simulink subsystem "darm_mechanics"  (R2021a)
settings: Solver=VariableStepAuto  StartTime=0.0  StopTime=10.0  RelTol=1e-3
undefined symbols (not defined in the file): darm, darm_knm, X, Y, Z
libraries: sm_lib x97, darm_library x77
(part 1 of 5)
settings Model: Creator=Daniel Adejumo  LastModifiedBy=Daniel Adejumo

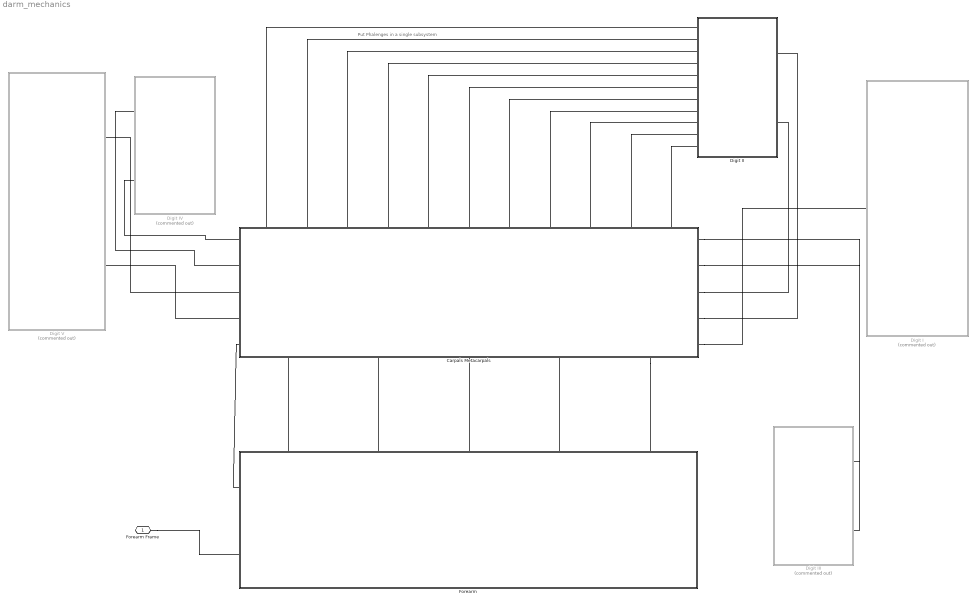
== system darm_mechanics ==
  note: Put Phalenges in a single subsystem
  Carpals Metacarpals : Subsystem
      settings: PortSchema="{\"entries\":[{\"content\":{\"sides\":[{\"content\":{\"connectorIds\":[\"LConn1\",\"LConn2\",\"LConn3\",\"LConn4\",\"LConn5\"]},\"type\":\"ConnectorPlacement.EquallySpacedRectSide\",\"uuid\":\"1bb88bb5-2f51-485d-a230-98e5c1753d25\"},{\"content\":{\"connectorIds\":[\"RConn1\",\"RConn2\",\"RConn3\",\"RConn4\",\"RConn5\"],\"side\":\"RIGHT\"},\"type\":\"ConnectorPlacement.EquallySpacedRectSide\",\"uuid\":\"55be408a-2070-4958-a81d-61010d6765a4\"},{\"content\":{\"connectorIds\":[\"LConn6\",\"LConn7\",\"LConn8\",\"LConn9\",\"LConn10\",\"LConn11\",\"LConn12\",\"LConn13\",\"LConn14\",\"LConn15\",\"LConn16\"],\"side\":\"TOP\"},\"type\":\"ConnectorPlacement.EquallySpacedRectSide\",\"uuid\":\"174f7df0-08cc-491e-9712-e123a58adeb3\"},{\"content\":{\"connectorIds\":[\"RConn6\",\"RConn7\",\"RConn8\",\"RConn9\",\"RConn10\"],\"side\":\"BOTTOM\"},\"type\":\"ConnectorPlacement.EquallySpacedRectSide\",\"uuid\":\"610f8ea9-4c2b-44d6-8efd-152cbdc7bfa9\"}]},\"type\":\"ConnectorPlacement.EquallySpacedConnector\",\"uuid\":\"f91d3c3d-350f-41e0-8fd3-766c28e2b75b\"}],\"packageUris\":[\"http://schema.mathworks.com/mf0/Connector/R2020b\"],\"version\":\"1.0\"}"
  Digit I : Subsystem  Commented=on
  Digit II : Subsystem
  Digit III : Subsystem  Commented=on
  Digit IV : Subsystem  Commented=on
  Digit V : Subsystem  Commented=on
  Forearm : Subsystem
      settings: PortSchema="{\"entries\":[{\"content\":{\"sides\":[{\"content\":{\"connectorIds\":[\"LConn1\",\"LConn2\"]},\"type\":\"ConnectorPlacement.EquallySpacedRectSide\",\"uuid\":\"5652e436-13d7-4977-ac7e-935b1a3f0729\"},{\"content\":{\"connectorIds\":[],\"side\":\"RIGHT\"},\"type\":\"ConnectorPlacement.EquallySpacedRectSide\",\"uuid\":\"721e98e9-19be-4402-ac40-382b694b4e6a\"},{\"content\":{\"connectorIds\":[\"LConn3\",\"LConn4\",\"LConn5\",\"LConn6\",\"LConn7\"],\"side\":\"TOP\"},\"type\":\"ConnectorPlacement.EquallySpacedRectSide\",\"uuid\":\"6b9e8076-ca0f-46eb-87d6-8c0e5d0c0dd4\"}]},\"type\":\"ConnectorPlacement.EquallySpacedConnector\",\"uuid\":\"9c8b8192-9cc9-4bae-a03f-e02120fb3373\"}],\"packageUris\":[\"http://schema.mathworks.com/mf0/Connector/R2020b\"],\"version\":\"1.0\"}"
  Forearm Frame : PMIOPort  Side=Left
  connections:
  Forearm Frame/RConn1 -- Forearm/LConn2
  Forearm/LConn1 -- Carpals Metacarpals/LConn5
  Carpals Metacarpals/RConn3 -- Digit II/RConn2
  Carpals Metacarpals/RConn4 -- Digit II/RConn1
  Carpals Metacarpals/RConn1 -- Digit III/RConn2
  Carpals Metacarpals/RConn2 -- Digit III/RConn1
  Carpals Metacarpals/LConn1 -- Digit IV/LConn2
  Carpals Metacarpals/LConn2 -- Digit IV/LConn1
  Carpals Metacarpals/LConn4 -- Digit V/RConn2
  Carpals Metacarpals/LConn3 -- Digit V/RConn1
  Carpals Metacarpals/RConn5 -- Digit I/RConn1
  Carpals Metacarpals/LConn6 -- Digit II/LConn1
  Carpals Metacarpals/LConn7 -- Digit II/LConn2
  Carpals Metacarpals/LConn8 -- Digit II/LConn3
  Carpals Metacarpals/LConn9 -- Digit II/LConn4
  Carpals Metacarpals/LConn10 -- Digit II/LConn5
  Carpals Metacarpals/LConn11 -- Digit II/LConn6
  Forearm/LConn3 -- Carpals Metacarpals/RConn6
  Forearm/LConn4 -- Carpals Metacarpals/RConn7
  Forearm/LConn5 -- Carpals Metacarpals/RConn8
  Carpals Metacarpals/LConn12 -- Digit II/LConn7
  Digit II/LConn8 -- Carpals Metacarpals/LConn13
  Carpals Metacarpals/LConn14 -- Digit II/LConn9
  Forearm/LConn6 -- Carpals Metacarpals/RConn9
  Carpals Metacarpals/LConn15 -- Digit II/LConn10
  Carpals Metacarpals/RConn10 -- Forearm/LConn7
  Carpals Metacarpals/LConn16 -- Digit II/LConn11

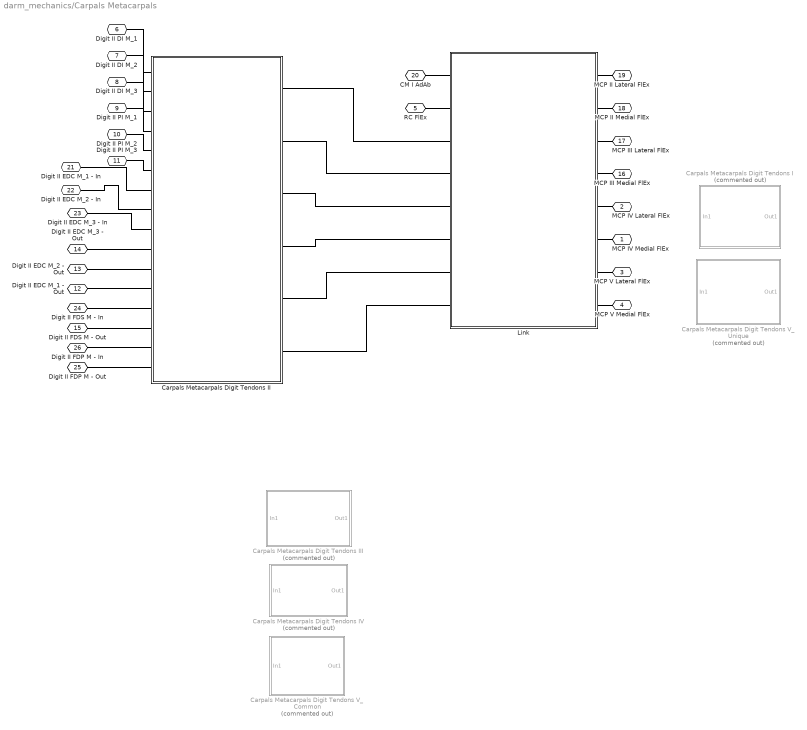
== system darm_mechanics/Carpals Metacarpals ==
  Carpals Metacarpals Digit Tendons I : Subsystem  Commented=on
  Carpals Metacarpals Digit Tendons II : Subsystem
  Carpals Metacarpals Digit Tendons III : Subsystem  Commented=on
  Carpals Metacarpals Digit Tendons IV : Subsystem  Commented=on
  Carpals Metacarpals Digit Tendons V_Common : Subsystem  Commented=on
  Carpals Metacarpals Digit Tendons V_Unique : Subsystem  Commented=on
  Link : Subsystem
  MCP IV Medial FlEx : PMIOPort  Side=Left
  MCP IV Lateral FlEx : PMIOPort  Port=2  Side=Left
  MCP V Lateral FlEx : PMIOPort  Port=3  Side=Left
  MCP V Medial FlEx : PMIOPort  Port=4  Side=Left
  RC FlEx : PMIOPort  Port=5  Side=Left
  Digit II DI M_1 : PMIOPort  Port=6  Side=Left
  Digit II DI M_2 : PMIOPort  Port=7  Side=Left
  Digit II DI M_3 : PMIOPort  Port=8  Side=Left
  Digit II PI M_1 : PMIOPort  Port=9  Side=Left
  Digit II PI M_2 : PMIOPort  Port=10  Side=Left
  Digit II PI M_3 : PMIOPort  Port=11  Side=Left
  Digit II EDC M_1 - Out : PMIOPort  Port=12  Side=Left
  Digit II EDC M_2 - Out : PMIOPort  Port=13  Side=Left
  Digit II EDC M_3 - Out : PMIOPort  Port=14  Side=Left
  Digit II FDS M - Out : PMIOPort  Port=15  Side=Left
  MCP III Medial FlEx : PMIOPort  Port=16  Side=Right
  MCP III Lateral FlEx : PMIOPort  Port=17  Side=Right
  MCP II Medial FlEx : PMIOPort  Port=18  Side=Right
  MCP II Lateral FlEx : PMIOPort  Port=19  Side=Right
  CM I AdAb : PMIOPort  Port=20  Side=Right
  Digit II EDC M_1 - In : PMIOPort  Port=21  Side=Right
  Digit II EDC M_2 - In : PMIOPort  Port=22  Side=Right
  Digit II EDC M_3 - In : PMIOPort  Port=23  Side=Right
  Digit II FDS M - In : PMIOPort  Port=24  Side=Right
  Digit II FDP M - Out : PMIOPort  Port=25  Side=Left
  Digit II FDP M - In : PMIOPort  Port=26  Side=Right
  connections:
  Digit II FDP M - In/RConn1 -- Carpals Metacarpals Digit Tendons II/LConn15
  Digit II FDP M - Out/RConn1 -- Carpals Metacarpals Digit Tendons II/LConn16
  Carpals Metacarpals Digit Tendons II/RConn6 -- Link/RConn8
  Carpals Metacarpals Digit Tendons II/RConn5 -- Link/RConn7
  Carpals Metacarpals Digit Tendons II/RConn4 -- Link/RConn6
  Digit II FDS M - Out/RConn1 -- Carpals Metacarpals Digit Tendons II/LConn14
  Digit II FDS M - In/RConn1 -- Carpals Metacarpals Digit Tendons II/LConn13
  Carpals Metacarpals Digit Tendons II/RConn3 -- Link/RConn5
  Digit II EDC M_1 - Out/RConn1 -- Carpals Metacarpals Digit Tendons II/LConn12
  Digit II EDC M_2 - Out/RConn1 -- Carpals Metacarpals Digit Tendons II/LConn11
  Digit II EDC M_3 - Out/RConn1 -- Carpals Metacarpals Digit Tendons II/LConn10
  Digit II EDC M_3 - In/RConn1 -- Carpals Metacarpals Digit Tendons II/LConn9
  Digit II EDC M_2 - In/RConn1 -- Carpals Metacarpals Digit Tendons II/LConn8
  Digit II EDC M_1 - In/RConn1 -- Carpals Metacarpals Digit Tendons II/LConn7
  Carpals Metacarpals Digit Tendons II/RConn2 -- Link/RConn4
  Digit II PI M_3/RConn1 -- Carpals Metacarpals Digit Tendons II/LConn6
  Digit II PI M_2/RConn1 -- Carpals Metacarpals Digit Tendons II/LConn5
  Digit II PI M_1/RConn1 -- Carpals Metacarpals Digit Tendons II/LConn4
  Digit II DI M_3/RConn1 -- Carpals Metacarpals Digit Tendons II/LConn3
  Digit II DI M_2/RConn1 -- Carpals Metacarpals Digit Tendons II/LConn2
  Digit II DI M_1/RConn1 -- Carpals Metacarpals Digit Tendons II/LConn1
  Carpals Metacarpals Digit Tendons II/RConn1 -- Link/RConn3
  CM I AdAb/RConn1 -- Link/RConn1
  Link/LConn8 -- MCP V Medial FlEx/RConn1
  Link/LConn7 -- MCP V Lateral FlEx/RConn1
  Link/LConn6 -- MCP IV Medial FlEx/RConn1
  Link/LConn5 -- MCP IV Lateral FlEx/RConn1
  Link/LConn4 -- MCP III Medial FlEx/RConn1
  Link/LConn3 -- MCP III Lateral FlEx/RConn1
  MCP II Medial FlEx/RConn1 -- Link/LConn2
  MCP II Lateral FlEx/RConn1 -- Link/LConn1
  RC FlEx/RConn1 -- Link/RConn2

== system darm_mechanics/Digit I ==
  Digit Links Assembly : Subsystem  AncestorBlock=darm_library/Digit Links Assembly  mask{digit=darm_knm.phalenges.digit_i}
      mask prompts: digit "Digit Struct"
      mask DialogControl DescGroupVar Prompt: Digit Links Assembly
      mask DialogControl DescTextVar Prompt: Assembles the phalanxes and joint shafts of a digit. Assembly spans from the proximal phalanx to the distal phalanx, excluding MCP Joint shafts.
  CM AdAb : PMIOPort  Side=Right
  connections:
  Digit Links Assembly/LConn4 -- CM AdAb/RConn1

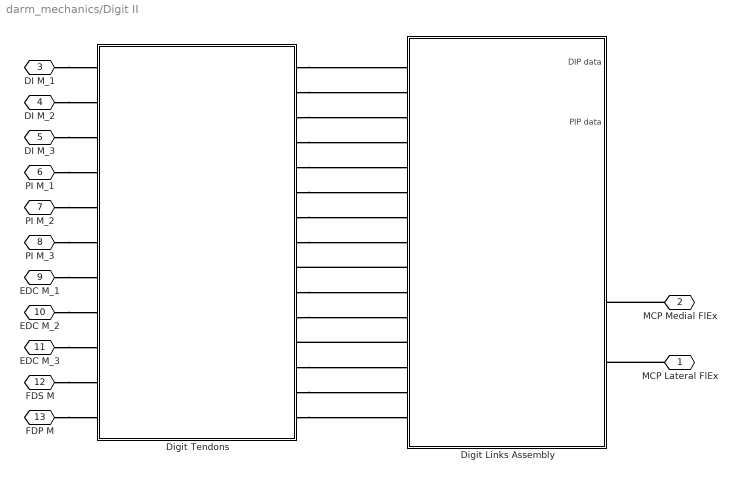
== system darm_mechanics/Digit II ==
  Digit Links Assembly : Subsystem  AncestorBlock=darm_library/Digit Links Assembly  mask{digit=darm.phalenges.digit_ii}
      mask prompts: digit "Digit Struct"
      mask DialogControl DescGroupVar Prompt: Digit Links Assembly
      mask DialogControl DescTextVar Prompt: Assembles the phalanxes and joint shafts of a digit. Assembly spans from the proximal phalanx to the distal phalanx, excluding MCP Joint shafts.
  Digit Tendons : Subsystem
  MCP Lateral FlEx : PMIOPort  Side=Right
  MCP Medial FlEx : PMIOPort  Port=2  Side=Right
  DI M_1 : PMIOPort  Port=3  Side=Left
  DI M_2 : PMIOPort  Port=4  Side=Left
  DI M_3 : PMIOPort  Port=5  Side=Left
  PI M_1 : PMIOPort  Port=6  Side=Left
  PI M_2 : PMIOPort  Port=7  Side=Left
  PI M_3 : PMIOPort  Port=8  Side=Left
  EDC M_1 : PMIOPort  Port=9  Side=Left
  EDC M_2 : PMIOPort  Port=10  Side=Left
  EDC M_3 : PMIOPort  Port=11  Side=Left
  FDS M : PMIOPort  Port=12  Side=Left
  FDP M : PMIOPort  Port=13  Side=Left
  connections:
  Digit Tendons/RConn15 -- Digit Links Assembly/LConn15
  Digit Tendons/RConn14 -- Digit Links Assembly/LConn14
  Digit Tendons/RConn1 -- Digit Links Assembly/LConn1
  FDP M/RConn1 -- Digit Tendons/LConn11
  Digit Tendons/RConn13 -- Digit Links Assembly/LConn13
  Digit Links Assembly/LConn12 -- Digit Tendons/RConn12
  FDS M/RConn1 -- Digit Tendons/LConn10
  Digit Tendons/RConn3 -- Digit Links Assembly/LConn3
  EDC M_3/RConn1 -- Digit Tendons/LConn9
  EDC M_2/RConn1 -- Digit Tendons/LConn8
  EDC M_1/RConn1 -- Digit Tendons/LConn7
  Digit Tendons/RConn8 -- Digit Links Assembly/LConn8
  Digit Tendons/RConn7 -- Digit Links Assembly/LConn7
  Digit Tendons/RConn11 -- Digit Links Assembly/LConn11
  PI M_3/RConn1 -- Digit Tendons/LConn6
  PI M_2/RConn1 -- Digit Tendons/LConn5
  PI M_1/RConn1 -- Digit Tendons/LConn4
  Digit Tendons/RConn10 -- Digit Links Assembly/LConn10
  Digit Links Assembly/LConn9 -- Digit Tendons/RConn9
  Digit Tendons/RConn5 -- Digit Links Assembly/LConn5
  DI M_3/RConn1 -- Digit Tendons/LConn3
  DI M_2/RConn1 -- Digit Tendons/LConn2
  Digit Tendons/RConn2 -- Digit Links Assembly/LConn2
  Digit Tendons/RConn4 -- Digit Links Assembly/LConn4
  DI M_1/RConn1 -- Digit Tendons/LConn1
  Digit Tendons/RConn6 -- Digit Links Assembly/LConn6
  MCP Lateral FlEx/RConn1 -- Digit Links Assembly/RConn4
  MCP Medial FlEx/RConn1 -- Digit Links Assembly/RConn3

== system darm_mechanics/Digit III ==
  Digit Links Assembly : Subsystem  AncestorBlock=darm_library/Digit Links Assembly  mask{digit=darm_knm.phalenges.digit_iii}
      mask prompts: digit "Digit Struct"
      mask DialogControl DescGroupVar Prompt: Digit Links Assembly
      mask DialogControl DescTextVar Prompt: Assembles the phalanxes and joint shafts of a digit. Assembly spans from the proximal phalanx to the distal phalanx, excluding MCP Joint shafts.
  MCP Lateral FlEx : PMIOPort  Side=Right
  MCP Medial FlEx : PMIOPort  Port=2  Side=Right
  connections:
  Digit Links Assembly/LConn4 -- MCP Lateral FlEx/RConn1
  Digit Links Assembly/LConn5 -- MCP Medial FlEx/RConn1

== system darm_mechanics/Digit IV ==
  Digit Links Assembly : Subsystem  AncestorBlock=darm_library/Digit Links Assembly  mask{digit=darm_knm.phalenges.digit_iv}
      mask prompts: digit "Digit Struct"
      mask DialogControl DescGroupVar Prompt: Digit Links Assembly
      mask DialogControl DescTextVar Prompt: Assembles the phalanxes and joint shafts of a digit. Assembly spans from the proximal phalanx to the distal phalanx, excluding MCP Joint shafts.
  MCP Lateral FlEx : PMIOPort  Side=Left
  MCP Medial FlEx : PMIOPort  Port=2  Side=Left
  connections:
  Digit Links Assembly/LConn4 -- MCP Lateral FlEx/RConn1
  Digit Links Assembly/LConn5 -- MCP Medial FlEx/RConn1

== system darm_mechanics/Digit V ==
  Digit Links Assembly : Subsystem  AncestorBlock=darm_library/Digit Links Assembly  mask{digit=darm_knm.phalenges.digit_v}
      mask prompts: digit "Digit Struct"
      mask DialogControl DescGroupVar Prompt: Digit Links Assembly
      mask DialogControl DescTextVar Prompt: Assembles the phalanxes and joint shafts of a digit. Assembly spans from the proximal phalanx to the distal phalanx, excluding MCP Joint shafts.
  MCP Lateral FlEx : PMIOPort  Side=Right
  MCP Medial FlEx : PMIOPort  Port=2  Side=Right
  connections:
  Digit Links Assembly/LConn5 -- MCP Medial FlEx/RConn1
  Digit Links Assembly/LConn4 -- MCP Lateral FlEx/RConn1

== system darm_mechanics/Forearm ==
  Forearm Digit Tendons II : Subsystem
  Link : Subsystem
  RC FlEx : PMIOPort  Side=Left
  Forearm Frame : PMIOPort  Port=2  Side=Left
  Digit II EDC M_1 : PMIOPort  Port=3  Side=Left
  Digit II EDC M_2 : PMIOPort  Port=4  Side=Left
  Digit II EDC M_3 : PMIOPort  Port=5  Side=Left
  Digit II FDS M : PMIOPort  Port=6  Side=Left
  Digit II FDP M : PMIOPort  Port=7  Side=Left
  connections:
  Digit II FDP M/RConn1 -- Forearm Digit Tendons II/LConn5
  Digit II FDS M/RConn1 -- Forearm Digit Tendons II/LConn4
  Digit II EDC M_1/RConn1 -- Forearm Digit Tendons II/LConn1
  Digit II EDC M_2/RConn1 -- Forearm Digit Tendons II/LConn2
  Digit II EDC M_3/RConn1 -- Forearm Digit Tendons II/LConn3
  Link/RConn1 -- Forearm Digit Tendons II/RConn1 -- RC FlEx/RConn1
  Forearm Digit Tendons II/RConn2 -- Forearm Frame/RConn1 -- Link/RConn2

== system darm_mechanics/Carpals Metacarpals/Carpals Metacarpals Digit Tendons I ==
  In1 : Inport
  Out1 : Outport
  wires:
  In1/1 -> Out1/1

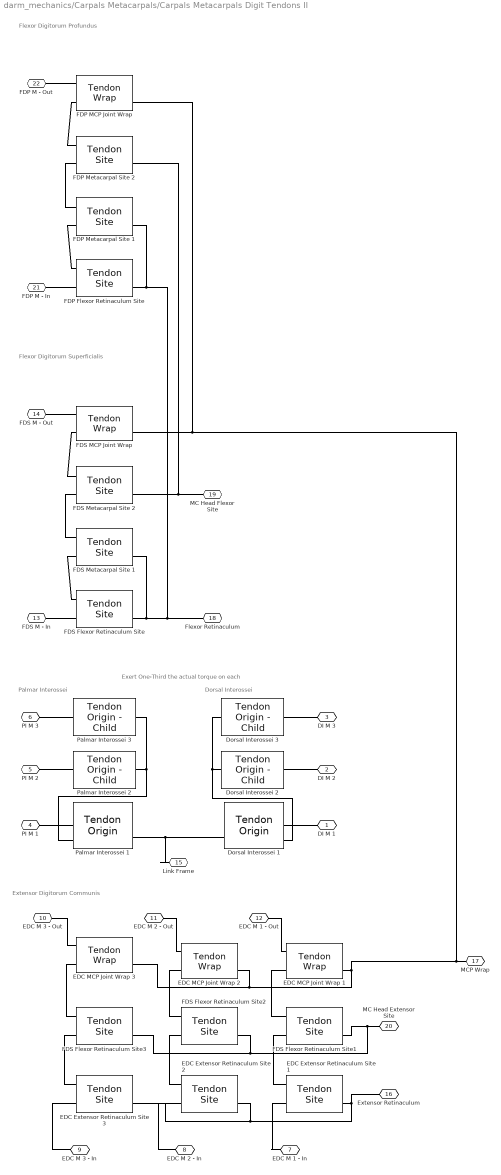
== system darm_mechanics/Carpals Metacarpals/Carpals Metacarpals Digit Tendons II ==
  note: Flexor Digitorum Profundus
  note: Palmar Interossei
  note: Exert One-Third the actual torque on each
  note: Dorsal Interossei
  note: Extensor Digitorum Communis
  note: Flexor Digitorum Superficialis
  Dorsal Interossei 1 : darm_library/Tendon Origin  muscle=darm.muscles.dorsal_interossei
  Dorsal Interossei 2 : darm_library/Tendon Origin - Child  muscle=darm.muscles.dorsal_interossei
  Dorsal Interossei 3 : darm_library/Tendon Origin - Child  muscle=darm.muscles.dorsal_interossei
  EDC Extensor Retinaculum Site 1 : darm_library/Tendon Site  muscle=darm.muscles.extensor_digitorum  site_index=1
  EDC Extensor Retinaculum Site 2 : darm_library/Tendon Site  muscle=darm.muscles.extensor_digitorum  site_index=1
  EDC Extensor Retinaculum Site 3 : darm_library/Tendon Site  muscle=darm.muscles.extensor_digitorum  site_index=1
  EDC MCP Joint Wrap 1 : darm_library/Tendon Wrap  muscle=darm.muscles.extensor_digitorum  wrap_index=2  flip=off
  EDC MCP Joint Wrap 2 : darm_library/Tendon Wrap  muscle=darm.muscles.extensor_digitorum  wrap_index=2  flip=off
  EDC MCP Joint Wrap 3 : darm_library/Tendon Wrap  muscle=darm.muscles.extensor_digitorum  wrap_index=2  flip=off
  FDP Flexor Retinaculum Site : darm_library/Tendon Site  muscle=darm.muscles.flexor_digitorum_profundus  site_index=1
  FDP MCP Joint Wrap : darm_library/Tendon Wrap  muscle=darm.muscles.flexor_digitorum_profundus  wrap_index=2  flip=on
  FDP Metacarpal Site 1 : darm_library/Tendon Site  muscle=darm.muscles.flexor_digitorum_profundus  site_index=3
  FDP Metacarpal Site 2 : darm_library/Tendon Site  muscle=darm.muscles.flexor_digitorum_profundus  site_index=5
  FDS Flexor Retinaculum Site : darm_library/Tendon Site  muscle=darm.muscles.flexor_digitorum_superficialis  site_index=1
  FDS Flexor Retinaculum Site1 : darm_library/Tendon Site  muscle=darm.muscles.extensor_digitorum  site_index=3
  FDS Flexor Retinaculum Site2 : darm_library/Tendon Site  muscle=darm.muscles.extensor_digitorum  site_index=3
  FDS Flexor Retinaculum Site3 : darm_library/Tendon Site  muscle=darm.muscles.extensor_digitorum  site_index=3
  FDS MCP Joint Wrap : darm_library/Tendon Wrap  muscle=darm.muscles.flexor_digitorum_superficialis  wrap_index=2  flip=on
  FDS Metacarpal Site 1 : darm_library/Tendon Site  muscle=darm.muscles.flexor_digitorum_superficialis  site_index=3
  FDS Metacarpal Site 2 : darm_library/Tendon Site  muscle=darm.muscles.flexor_digitorum_superficialis  site_index=5
  Palmar Interossei 1 : darm_library/Tendon Origin  muscle=darm.muscles.palmar_interossei
  Palmar Interossei 2 : darm_library/Tendon Origin - Child  muscle=darm.muscles.palmar_interossei
  Palmar Interossei 3 : darm_library/Tendon Origin - Child  muscle=darm.muscles.palmar_interossei
  DI M 1 : PMIOPort  Side=Left
  DI M 2 : PMIOPort  Port=2  Side=Left
  DI M 3 : PMIOPort  Port=3  Side=Left
  PI M 1 : PMIOPort  Port=4  Side=Left
  PI M 2 : PMIOPort  Port=5  Side=Left
  PI M 3 : PMIOPort  Port=6  Side=Left
  EDC M 1 - In : PMIOPort  Port=7  Side=Left
  EDC M 2 - In : PMIOPort  Port=8  Side=Left
  EDC M 3 - In : PMIOPort  Port=9  Side=Left
  EDC M 3 - Out : PMIOPort  Port=10  Side=Left
  EDC M 2 - Out : PMIOPort  Port=11  Side=Left
  EDC M 1 - Out : PMIOPort  Port=12  Side=Left
  FDS M - In : PMIOPort  Port=13  Side=Left
  FDS M - Out : PMIOPort  Port=14  Side=Left
  Link Frame : PMIOPort  Port=15  Side=Right
  Extensor Retinaculum : PMIOPort  Port=16  Side=Right
  MCP Wrap : PMIOPort  Port=17  Side=Right
  Flexor Retinaculum : PMIOPort  Port=18  Side=Right
  MC Head Flexor Site : PMIOPort  Port=19  Side=Right
  MC Head Extensor Site : PMIOPort  Port=20  Side=Right
  FDP M - In : PMIOPort  Port=21  Side=Left
  FDP M - Out : PMIOPort  Port=22  Side=Left
  connections:
  Dorsal Interossei 3/RConn1 -- Dorsal Interossei 2/RConn1 -- Dorsal Interossei 1/RConn2
  Palmar Interossei 3/RConn1 -- Palmar Interossei 2/RConn1 -- Palmar Interossei 1/RConn2
  FDP Metacarpal Site 1/LConn2 -- FDP Flexor Retinaculum Site/LConn1
  FDP Metacarpal Site 2/LConn1 -- FDP MCP Joint Wrap/LConn2
  FDP M - In/RConn1 -- FDP Flexor Retinaculum Site/LConn2
  FDP M - Out/RConn1 -- FDP MCP Joint Wrap/LConn1
  FDP Metacarpal Site 1/LConn1 -- FDP Metacarpal Site 2/LConn2
  FDS Flexor Retinaculum Site3/LConn1 -- EDC MCP Joint Wrap 3/LConn2
  FDS Flexor Retinaculum Site2/LConn1 -- EDC MCP Joint Wrap 2/LConn2
  FDS Flexor Retinaculum Site1/LConn1 -- EDC MCP Joint Wrap 1/LConn2
  EDC Extensor Retinaculum Site 1/LConn1 -- FDS Flexor Retinaculum Site1/LConn2
  FDS Flexor Retinaculum Site3/RConn1 -- MC Head Extensor Site/RConn1 -- FDS Flexor Retinaculum Site1/RConn1 -- FDS Flexor Retinaculum Site2/RConn1
  FDP Metacarpal Site 2/RConn1 -- MC Head Flexor Site/RConn1 -- FDS Metacarpal Site 2/RConn1
  FDS Metacarpal Site 2/LConn1 -- FDS MCP Joint Wrap/LConn2
  FDS Metacarpal Site 1/LConn1 -- FDS Metacarpal Site 2/LConn2
  FDP Flexor Retinaculum Site/RConn1 -- FDP Metacarpal Site 1/RConn1 -- Flexor Retinaculum/RConn1 -- FDS Flexor Retinaculum Site/RConn1 -- FDS Metacarpal Site 1/RConn1
  FDS M - Out/RConn1 -- FDS MCP Joint Wrap/LConn1
  FDS M - In/RConn1 -- FDS Flexor Retinaculum Site/LConn2
  FDS Metacarpal Site 1/LConn2 -- FDS Flexor Retinaculum Site/LConn1
  FDS Flexor Retinaculum Site3/LConn2 -- EDC Extensor Retinaculum Site 3/LConn1
  EDC M 3 - Out/RConn1 -- EDC MCP Joint Wrap 3/LConn1
  EDC Extensor Retinaculum Site 2/LConn1 -- FDS Flexor Retinaculum Site2/LConn2
  EDC M 2 - Out/RConn1 -- EDC MCP Joint Wrap 2/LConn1
  EDC M 1 - Out/RConn1 -- EDC MCP Joint Wrap 1/LConn1
  FDP MCP Joint Wrap/RConn1 -- FDS MCP Joint Wrap/RConn1 -- MCP Wrap/RConn1 -- EDC MCP Joint Wrap 1/RConn1 -- EDC MCP Joint Wrap 3/RConn1 -- EDC MCP Joint Wrap 2/RConn1
  EDC M 2 - In/RConn1 -- EDC Extensor Retinaculum Site 2/LConn2
  EDC M 1 - In/RConn1 -- EDC Extensor Retinaculum Site 1/LConn2
  EDC M 3 - In/RConn1 -- EDC Extensor Retinaculum Site 3/LConn2
  EDC Extensor Retinaculum Site 2/RConn1 -- EDC Extensor Retinaculum Site 3/RConn1 -- EDC Extensor Retinaculum Site 1/RConn1 -- Extensor Retinaculum/RConn1
  PI M 1/RConn1 -- Palmar Interossei 1/RConn1
  PI M 2/RConn1 -- Palmar Interossei 2/LConn1
  Palmar Interossei 3/LConn1 -- PI M 3/RConn1
  DI M 3/RConn1 -- Dorsal Interossei 3/LConn1
  DI M 2/RConn1 -- Dorsal Interossei 2/LConn1
  DI M 1/RConn1 -- Dorsal Interossei 1/RConn1
  Dorsal Interossei 1/LConn1 -- Palmar Interossei 1/LConn1 -- Link Frame/RConn1

== system darm_mechanics/Carpals Metacarpals/Carpals Metacarpals Digit Tendons III ==
  In1 : Inport
  Out1 : Outport
  wires:
  In1/1 -> Out1/1

== system darm_mechanics/Carpals Metacarpals/Carpals Metacarpals Digit Tendons IV ==
  In1 : Inport
  Out1 : Outport
  wires:
  In1/1 -> Out1/1

== system darm_mechanics/Carpals Metacarpals/Carpals Metacarpals Digit Tendons V_Common ==
  In1 : Inport
  Out1 : Outport
  wires:
  In1/1 -> Out1/1

== system darm_mechanics/Carpals Metacarpals/Carpals Metacarpals Digit Tendons V_Unique ==
  In1 : Inport
  Out1 : Outport
  wires:
  In1/1 -> Out1/1

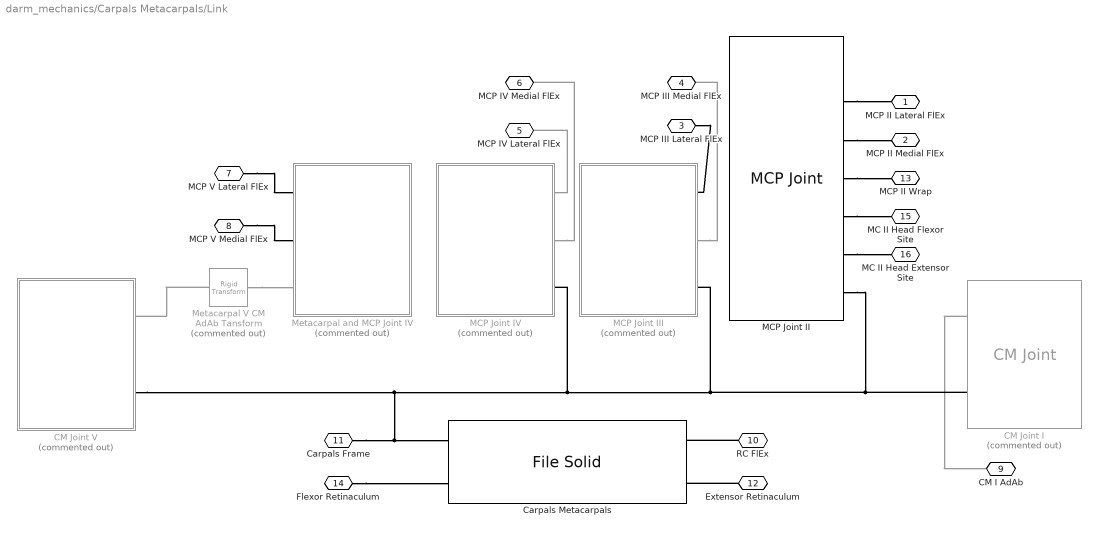
== system darm_mechanics/Carpals Metacarpals/Link ==
  CM Joint I : darm_library/CM Joint  Commented=on  cm=darm_knm.carpals.cm_i
  CM Joint V : Subsystem  Commented=on  AncestorBlock=darm_library/CM Joint  mask{cm=darm_knm.carpals.cm_v}
      mask prompts: cm "CM Struct"
      mask DialogControl DescGroupVar Prompt: Carpometacarpal Joint
      mask DialogControl DescTextVar Prompt: Models the centre block, flexion/extension and adduction/abduction joints, and the transform from the carpals frame.
  Carpals Metacarpals : sm_lib/Body Elements/File Solid  ExtGeomFileName=C:\Users\Daniel Adejumo\Documents\MATLAB\DARM\Geometry Models and FEA\Models\CAD\Carpals Metacarpals\Carpals Base.step  UnitType=FromFile  ExtGeomFileUnits=m  StepReaderType=HEX  ExportConvexHullGeometry=off  InertiaType=CalculateFromGeometry  Mass=1  MassUnits=kg  CenterOfMass=[0 0 0]  CenterOfMassUnits=m  MomentsOfInertia=[1 1 1]  MomentsOfInertiaUnits=kg*m^2  ProductsOfInertia=[0 0 0]  ProductsOfInertiaUnits=kg*m^2  BasedOnType=Density  Density=darm.link_density  DensityUnits=kg/m^3  DoExposeReferenceFrame=on  SerializedFrames=<Frames><Frame><Id>Frame1</Id><Value><Name>J</Name><Origin><Source>ReferenceFrame</Source><FeatureName></FeatureName></Origin><PrimaryAxis><DefinedDirection>+Z</DefinedDirection><Source>ReferenceFrame</Source><SourceDirection>+X</SourceDirection><FeatureName></FeatureName></PrimaryAxis><SecondaryAxis><DefinedDirection>+X</DefinedDirection><Source>ReferenceFrame</Source><SourceDirection>-Z</SourceDirection><FeatureName></FeatureName></SecondaryAxis></Value></Frame><Frame><Id>Frame2</Id><Value><Name>Extensor Retinaculum</Name><Origin><Source>GeometricFeature</Source><FeatureName>segment 10</FeatureName></Origin><PrimaryAxis><DefinedDirection>+Z</DefinedDirection><Source>ReferenceFrame</Source><SourceDirection>+Z</SourceDirection><FeatureName></FeatureName></PrimaryAxis><SecondaryAxis><DefinedDirection>+X</DefinedDirection><Source>ReferenceFrame</Source><SourceDirection>+X</SourceDirection><FeatureName></FeatureName></SecondaryAxis></Value></Frame><Frame><Id>Frame3</Id><Value><Name>Flexor Retinaculum</Name><Origin><Source>GeometricFeature</Source><FeatureName>segment 8</FeatureName></Origin><PrimaryAxis><DefinedDirection>+Z</DefinedDirection><Source>ReferenceFrame</Source><SourceDirection>+Z</SourceDirection><FeatureName></FeatureName></PrimaryAxis><SecondaryAxis><DefinedDirection>+X</DefinedDirection><Source>ReferenceFrame</Source><SourceDirection>+X</SourceDirection><FeatureName></FeatureName></SecondaryAxis></Value></Frame></Frames>  GraphicType=FromGeometry  MarkerShape=Sphere  MarkerSize=10  GraphicVisPropType=SimpleVisualProperties  GraphicDiffuseColor=[0.5 0.5 0.5]  GraphicSpecularColor=[0.5 0.5 0.5 1.0]  GraphicAmbientColor=[0.15 0.15 0.15 1.0]  GraphicEmissiveColor=[0.0 0.0 0.0 1.0]  GraphicShininess=75  GraphicOpacity=1.0
  MCP Joint II : darm_library/MCP Joint  mcp=darm.carpals.mcp_ii
  MCP Joint III : Subsystem  Commented=on  AncestorBlock=darm_library/MCP Joint  mask{mcp=darm_knm.carpals.mcp_iii}
      mask prompts: mcp "MCP Struct"
      mask DialogControl DescGroupVar Prompt: Metacarpophalangeal Joint
      mask DialogControl DescTextVar Prompt: Models the centre block, flexion/extension and adduction/abduction joints, and the transform from the carpals frame.
  MCP Joint IV : Subsystem  Commented=on  AncestorBlock=darm_library/MCP Joint  mask{mcp=darm_knm.carpals.mcp_iv}
      mask prompts: mcp "MCP Struct"
      mask DialogControl DescGroupVar Prompt: Metacarpophalangeal Joint
      mask DialogControl DescTextVar Prompt: Models the centre block, flexion/extension and adduction/abduction joints, and the transform from the carpals frame.
  Metacarpal V CM AdAb Tansform : sm_lib/Frames and Transforms/Rigid Transform  Commented=on  TranslationMethod=StandardAxis  TranslationStandardOffset=darm_knm.carpals.cm_v.cm_joint_block_adab_thickness/2  TranslationLengthUnit=m  TranslationStandardAxis=+Z  TranslationCartesianOffset=[0 0 0]  TranslationROffset=0  TranslationROffsetUnits=m  TranslationZOffset=0  TranslationZOffsetUnits=m  TranslationThetaOffset=0  TranslationThetaOffsetUnits=deg  RotationMethod=None  RotationAngleUnits=deg  RotationStandardAxis=+Z  RotationAngle=0.0  RotationArbitraryAxis=[0 0 1]  FollAlignAxisA=+X  BaseAlignAxisA=+Y  FollAlignAxisB=+Y  BaseAlignAxisB=+Z  RotationSequenceAxes=FollowerAxes  RotationSequence=XYX  RotationSequenceAngles=[0 0 0]  RotationSequenceAnglesUnits=deg  RotationMatrix=[1 0 0; 0 1 0; 0 0 1]
  Metacarpal and MCP Joint IV : Subsystem  Commented=on  AncestorBlock=darm_library/MCP Joint  mask{mcp=darm_knm.carpals.mcp_v}
      mask prompts: mcp "MCP Struct"
      mask DialogControl DescGroupVar Prompt: Metacarpophalangeal Joint
      mask DialogControl DescTextVar Prompt: Models the centre block, flexion/extension and adduction/abduction joints, and the transform from the carpals frame.
  MCP II Lateral FlEx : PMIOPort  Side=Left
  MCP II Medial FlEx : PMIOPort  Port=2  Side=Left
  MCP III Lateral FlEx : PMIOPort  Port=3  Side=Left
  MCP III Medial FlEx : PMIOPort  Port=4  Side=Left
  MCP IV Lateral FlEx : PMIOPort  Port=5  Side=Left
  MCP IV Medial FlEx : PMIOPort  Port=6  Side=Left
  MCP V Lateral FlEx : PMIOPort  Port=7  Side=Left
  MCP V Medial FlEx : PMIOPort  Port=8  Side=Left
  CM I AdAb : PMIOPort  Port=9  Side=Right
  RC FlEx : PMIOPort  Port=10  Side=Right
  Carpals Frame : PMIOPort  Port=11  Side=Right
  Extensor Retinaculum : PMIOPort  Port=12  Side=Right
  MCP II Wrap : PMIOPort  Port=13  Side=Right
  Flexor Retinaculum : PMIOPort  Port=14  Side=Right
  MC II Head Flexor Site : PMIOPort  Port=15  Side=Right
  MC II Head Extensor Site : PMIOPort  Port=16  Side=Right
  connections:
  MCP Joint II/RConn5 -- MC II Head Extensor Site/RConn1
  MCP Joint II/RConn4 -- MC II Head Flexor Site/RConn1
  MCP Joint II/RConn3 -- MCP II Wrap/RConn1
  Flexor Retinaculum/RConn1 -- Carpals Metacarpals/RConn2
  Extensor Retinaculum/RConn1 -- Carpals Metacarpals/LConn2
  MCP Joint IV/RConn2 -- MCP IV Medial FlEx/RConn1
  MCP Joint IV/RConn1 -- MCP IV Lateral FlEx/RConn1
  MCP V Medial FlEx/RConn1 -- Metacarpal and MCP Joint IV/RConn2
  MCP V Lateral FlEx/RConn1 -- Metacarpal and MCP Joint IV/RConn1
  MCP Joint III/RConn2 -- MCP III Medial FlEx/RConn1
  MCP III Lateral FlEx/RConn1 -- MCP Joint III/RConn1
  Metacarpal V CM AdAb Tansform/RConn1 -- CM Joint V/LConn1
  Metacarpal V CM AdAb Tansform/LConn1 -- Metacarpal and MCP Joint IV/RConn3
  CM Joint I/LConn1 -- CM I AdAb/RConn1
  MCP Joint II/RConn2 -- MCP II Medial FlEx/RConn1
  MCP Joint II/RConn1 -- MCP II Lateral FlEx/RConn1
  MCP Joint II/RConn6 -- CM Joint I/LConn2 -- MCP Joint IV/RConn3 -- Carpals Metacarpals/RConn1 -- Carpals Frame/RConn1 -- CM Joint V/LConn2 -- MCP Joint III/RConn3
  RC FlEx/RConn1 -- Carpals Metacarpals/LConn1

== system darm_mechanics/Digit I/Digit Links Assembly ==
  DIP Joint Shaft : sm_lib/Body Elements/Cylindrical Solid  GraphicAmbientColor=[0.15 0.15 0.15 1.0]  BasedOnType=Density  CenterOfMass=[0 0 0]  CenterOfMassUnits=m  GraphicDiffuseColor=[0.5 0.5 0.5]  CylinderLength=digit.dip_joint_shaft_length  CylinderLengthUnits=m  CylinderRadius=digit.dip_joint_shaft_radius  CylinderRadiusUnits=m  Density=darm_dnm.link_density  DensityUnits=kg/m^3  DoExposeReferenceFrame=on  GraphicEmissiveColor=[0.0 0.0 0.0 1.0]  ExportEntireGeometry=off  SerializedFrames=<Frames/>  MarkerShape=Sphere  MarkerSize=10  GraphicType=FromGeometry  InertiaType=CalculateFromGeometry  Mass=1  MassUnits=kg  MomentsOfInertia=[1 1 1]  MomentsOfInertiaUnits=kg*m^2  GraphicOpacity=1.0  ProductsOfInertia=[0 0 0]  ProductsOfInertiaUnits=kg*m^2  GraphicShininess=75  GraphicSpecularColor=[0.5 0.5 0.5 1.0]  GraphicVisPropType=SimpleVisualProperties
  Distal Phalanx : sm_lib/Body Elements/File Solid  ExtGeomFileName=Geometry Models and FEA\Models\CAD\Phalanges\Phalanges I\Distal Phalanx I.step  UnitType=FromFile  ExtGeomFileUnits=m  StepReaderType=HEX  ExportConvexHullGeometry=off  InertiaType=CalculateFromGeometry  Mass=1  MassUnits=kg  CenterOfMass=[0 0 0]  CenterOfMassUnits=m  MomentsOfInertia=[1 1 1]  MomentsOfInertiaUnits=kg*m^2  ProductsOfInertia=[0 0 0]  ProductsOfInertiaUnits=kg*m^2  BasedOnType=Density  Density=darm_dnm.link_density  DensityUnits=kg/m^3  DoExposeReferenceFrame=on  SerializedFrames=<Frames><Frame><Id>Frame1</Id><Value><Name>J</Name><Origin><Source>ReferenceFrame</Source><FeatureName></FeatureName></Origin><PrimaryAxis><DefinedDirection>+Z</DefinedDirection><Source>ReferenceFrame</Source><SourceDirection>+X</SourceDirection><FeatureName></FeatureName></PrimaryAxis><SecondaryAxis><DefinedDirection>+X</DefinedDirection><Source>ReferenceFrame</Source><SourceDirection>-Z</SourceDirection><FeatureName></FeatureName></SecondaryAxis></Value></Frame></Frames>  GraphicType=FromGeometry  MarkerShape=Sphere  MarkerSize=10  GraphicVisPropType=SimpleVisualProperties  GraphicDiffuseColor=[0.5 0.5 0.5]  GraphicSpecularColor=[0.5 0.5 0.5 1.0]  GraphicAmbientColor=[0.15 0.15 0.15 1.0]  GraphicEmissiveColor=[0.0 0.0 0.0 1.0]  GraphicShininess=75  GraphicOpacity=1.0
  Middle Phalanx : sm_lib/Body Elements/File Solid  ExtGeomFileName=Geometry Models and FEA\Models\CAD\Phalanges\Phalanges I\Proximal Phalanx I.step  UnitType=FromFile  ExtGeomFileUnits=m  StepReaderType=HEX  ExportConvexHullGeometry=off  InertiaType=CalculateFromGeometry  Mass=1  MassUnits=kg  CenterOfMass=[0 0 0]  CenterOfMassUnits=m  MomentsOfInertia=[1 1 1]  MomentsOfInertiaUnits=kg*m^2  ProductsOfInertia=[0 0 0]  ProductsOfInertiaUnits=kg*m^2  BasedOnType=Density  Density=darm_dnm.link_density  DensityUnits=kg/m^3  DoExposeReferenceFrame=on  SerializedFrames=<Frames><Frame><Id>Frame2</Id><Value><Name>DIP J*</Name><Origin><Source>GeometricFeature</Source><FeatureName>circular curve 222</FeatureName></Origin><PrimaryAxis><DefinedDirection>+Z</DefinedDirection><Source>ReferenceFrame</Source><SourceDirection>+X</SourceDirection><FeatureName></FeatureName></PrimaryAxis><SecondaryAxis><DefinedDirection>+X</DefinedDirection><Source>ReferenceFrame</Source><SourceDirection>-Z</SourceDirection><FeatureName></FeatureName></SecondaryAxis></Value></Frame><Frame><Id>Frame3</Id><Value><Name>PIP J</Name><Origin><Source>ReferenceFrame</Source><FeatureName></FeatureName></Origin><PrimaryAxis><DefinedDirection>+Z</DefinedDirection><Source>ReferenceFrame</Source><SourceDirection>+X</SourceDirection><FeatureName></FeatureName></PrimaryAxis><SecondaryAxis><DefinedDirection>+X</DefinedDirection><Source>ReferenceFrame</Source><SourceDirection>-Z</SourceDirection><FeatureName></FeatureName></SecondaryAxis></Value></Frame></Frames>  GraphicType=FromGeometry  MarkerShape=Sphere  MarkerSize=10  GraphicVisPropType=SimpleVisualProperties  GraphicDiffuseColor=[0.5 0.5 0.5]  GraphicSpecularColor=[0.5 0.5 0.5 1.0]  GraphicAmbientColor=[0.15 0.15 0.15 1.0]  GraphicEmissiveColor=[0.0 0.0 0.0 1.0]  GraphicShininess=75  GraphicOpacity=1.0
  PIP Joint Shaft : sm_lib/Body Elements/Cylindrical Solid  GraphicAmbientColor=[0.15 0.15 0.15 1.0]  BasedOnType=Density  CenterOfMass=[0 0 0]  CenterOfMassUnits=m  GraphicDiffuseColor=[0.5 0.5 0.5]  CylinderLength=digit.pip_joint_shaft_length  CylinderLengthUnits=m  CylinderRadius=digit.pip_joint_shaft_radius  CylinderRadiusUnits=m  Density=darm_dnm.link_density  DensityUnits=kg/m^3  DoExposeReferenceFrame=on  GraphicEmissiveColor=[0.0 0.0 0.0 1.0]  ExportEntireGeometry=off  SerializedFrames=<Frames/>  MarkerShape=Sphere  MarkerSize=10  GraphicType=FromGeometry  InertiaType=CalculateFromGeometry  Mass=1  MassUnits=kg  MomentsOfInertia=[1 1 1]  MomentsOfInertiaUnits=kg*m^2  GraphicOpacity=1.0  ProductsOfInertia=[0 0 0]  ProductsOfInertiaUnits=kg*m^2  GraphicShininess=75  GraphicSpecularColor=[0.5 0.5 0.5 1.0]  GraphicVisPropType=SimpleVisualProperties
  Proximal Phalanx : sm_lib/Body Elements/File Solid  ExtGeomFileName=C:\Users\Daniel Adejumo\Documents\MATLAB\DARM\Geometry Models and FEA\Models\CAD\Carpals Metacarpals\Metacarpal I\Metacarpal I.step  UnitType=FromFile  ExtGeomFileUnits=m  StepReaderType=HEX  ExportConvexHullGeometry=off  InertiaType=CalculateFromGeometry  Mass=1  MassUnits=kg  CenterOfMass=[0 0 0]  CenterOfMassUnits=m  MomentsOfInertia=[1 1 1]  MomentsOfInertiaUnits=kg*m^2  ProductsOfInertia=[0 0 0]  ProductsOfInertiaUnits=kg*m^2  BasedOnType=Density  Density=darm_dnm.link_density  DensityUnits=kg/m^3  DoExposeReferenceFrame=on  SerializedFrames=<Frames><Frame><Id>Frame1</Id><Value><Name>MCP J*</Name><Origin><Source>GeometricFeature</Source><FeatureName>circular curve 166</FeatureName></Origin><PrimaryAxis><DefinedDirection>+Z</DefinedDirection><Source>ReferenceFrame</Source><SourceDirection>+X</SourceDirection><FeatureName></FeatureName></PrimaryAxis><SecondaryAxis><DefinedDirection>+X</DefinedDirection><Source>ReferenceFrame</Source><SourceDirection>-Z</SourceDirection><FeatureName></FeatureName></SecondaryAxis></Value></Frame><Frame><Id>Frame2</Id><Value><Name>CM J</Name><Origin><Source>ReferenceFrame</Source><FeatureName></FeatureName></Origin><PrimaryAxis><DefinedDirection>+Z</DefinedDirection><Source>ReferenceFrame</Source><SourceDirection>+Y</SourceDirection><FeatureName></FeatureName></PrimaryAxis><SecondaryAxis><DefinedDirection>+X</DefinedDirection><Source>ReferenceFrame</Source><SourceDirection>+X</SourceDirection><FeatureName></FeatureName></SecondaryAxis></Value></Frame></Frames>  GraphicType=FromGeometry  MarkerShape=Sphere  MarkerSize=10  GraphicVisPropType=SimpleVisualProperties  GraphicDiffuseColor=[0.5 0.5 0.5]  GraphicSpecularColor=[0.5 0.5 0.5 1.0]  GraphicAmbientColor=[0.15 0.15 0.15 1.0]  GraphicEmissiveColor=[0.0 0.0 0.0 1.0]  GraphicShininess=75  GraphicOpacity=1.0
  Revolute Joint : sm_lib/Joints/Revolute Joint  JointMode=Normal  SenseConstraintForce=off  SenseConstraintForceX=off  SenseConstraintForceY=off  SenseConstraintForceZ=off  SenseConstraintTorque=off  SenseConstraintTorqueX=off  SenseConstraintTorqueY=off  SenseConstraintTorqueZ=off  SenseTotalForce=off  SenseTotalForceX=off  SenseTotalForceY=off  SenseTotalForceZ=off  SenseTotalTorque=off  SenseTotalTorqueX=off  SenseTotalTorqueY=off  SenseTotalTorqueZ=off  CompositeWrenchDir=FollowerOnBase  CompositeWrenchFrame=BaseFrame  EquilibriumPosition=0  EquilibriumPositionUnits=deg  SpringStiffness=0  SpringStiffnessUnits=N*m/deg  DampingCoefficient=0  DampingCoefficientUnits=N*m/(deg/s)  TorqueActuationMode=NoTorque  MotionActuationMode=ComputedMotion  SensePosition=off  SenseVelocity=off  SenseAcceleration=off  SenseTorqueForce=off  SenseLowerLimitTorqueForce=off  SenseUpperLimitTorqueForce=off  LowerLimitSpecify=off  LowerLimitBound=-90  LowerLimitBoundUnits=deg  LowerLimitStiffness=1e4  LowerLimitStiffnessUnits=N*m/deg  LowerLimitDamping=10  LowerLimitDampingUnits=N*m/(deg/s)  LowerLimitTransitionRegionWidth=0.1  LowerLimitTransitionRegionWidthUnits=deg  UpperLimitSpecify=off  UpperLimitBound=90  UpperLimitBoundUnits=deg  UpperLimitStiffness=1e4  UpperLimitStiffnessUnits=N*m/deg  UpperLimitDamping=10  UpperLimitDampingUnits=N*m/(deg/s)  UpperLimitTransitionRegionWidth=0.1  UpperLimitTransitionRegionWidthUnits=deg  PositionTargetSpecify=off  PositionTargetPriority=High  PositionTargetValue=0  PositionTargetValueUnits=deg  VelocityTargetSpecify=off  VelocityTargetPriority=High  VelocityTargetValue=0  VelocityTargetValueUnits=deg/s
  Revolute Joint1 : sm_lib/Joints/Revolute Joint  JointMode=Normal  SenseConstraintForce=off  SenseConstraintForceX=off  SenseConstraintForceY=off  SenseConstraintForceZ=off  SenseConstraintTorque=off  SenseConstraintTorqueX=off  SenseConstraintTorqueY=off  SenseConstraintTorqueZ=off  SenseTotalForce=off  SenseTotalForceX=off  SenseTotalForceY=off  SenseTotalForceZ=off  SenseTotalTorque=off  SenseTotalTorqueX=off  SenseTotalTorqueY=off  SenseTotalTorqueZ=off  CompositeWrenchDir=FollowerOnBase  CompositeWrenchFrame=BaseFrame  EquilibriumPosition=0  EquilibriumPositionUnits=deg  SpringStiffness=0  SpringStiffnessUnits=N*m/deg  DampingCoefficient=0  DampingCoefficientUnits=N*m/(deg/s)  TorqueActuationMode=NoTorque  MotionActuationMode=ComputedMotion  SensePosition=off  SenseVelocity=off  SenseAcceleration=off  SenseTorqueForce=off  SenseLowerLimitTorqueForce=off  SenseUpperLimitTorqueForce=off  LowerLimitSpecify=off  LowerLimitBound=-90  LowerLimitBoundUnits=deg  LowerLimitStiffness=1e4  LowerLimitStiffnessUnits=N*m/deg  LowerLimitDamping=10  LowerLimitDampingUnits=N*m/(deg/s)  LowerLimitTransitionRegionWidth=0.1  LowerLimitTransitionRegionWidthUnits=deg  UpperLimitSpecify=off  UpperLimitBound=90  UpperLimitBoundUnits=deg  UpperLimitStiffness=1e4  UpperLimitStiffnessUnits=N*m/deg  UpperLimitDamping=10  UpperLimitDampingUnits=N*m/(deg/s)  UpperLimitTransitionRegionWidth=0.1  UpperLimitTransitionRegionWidthUnits=deg  PositionTargetSpecify=off  PositionTargetPriority=High  PositionTargetValue=0  PositionTargetValueUnits=deg  VelocityTargetSpecify=off  VelocityTargetPriority=High  VelocityTargetValue=0  VelocityTargetValueUnits=deg/s
  Rigid Transform : sm_lib/Frames and Transforms/Rigid Transform  TranslationMethod=StandardAxis  TranslationStandardOffset=digit.dip_joint_length/4  TranslationLengthUnit=m  TranslationStandardAxis=+Z  TranslationCartesianOffset=[0 0 0]  TranslationROffset=0  TranslationROffsetUnits=m  TranslationZOffset=0  TranslationZOffsetUnits=m  TranslationThetaOffset=0  TranslationThetaOffsetUnits=deg  RotationMethod=None  RotationAngleUnits=deg  RotationStandardAxis=+Z  RotationAngle=0.0  RotationArbitraryAxis=[0 0 1]  FollAlignAxisA=+X  BaseAlignAxisA=+Y  FollAlignAxisB=+Y  BaseAlignAxisB=+Z  RotationSequenceAxes=FollowerAxes  RotationSequence=XYX  RotationSequenceAngles=[0 0 0]  RotationSequenceAnglesUnits=deg  RotationMatrix=[1 0 0; 0 1 0; 0 0 1]
  Rigid Transform1 : sm_lib/Frames and Transforms/Rigid Transform  TranslationMethod=StandardAxis  TranslationStandardOffset=digit.pip_joint_length/4  TranslationLengthUnit=m  TranslationStandardAxis=+Z  TranslationCartesianOffset=[0 0 0]  TranslationROffset=0  TranslationROffsetUnits=m  TranslationZOffset=0  TranslationZOffsetUnits=m  TranslationThetaOffset=0  TranslationThetaOffsetUnits=deg  RotationMethod=None  RotationAngleUnits=deg  RotationStandardAxis=+Z  RotationAngle=0.0  RotationArbitraryAxis=[0 0 1]  FollAlignAxisA=+X  BaseAlignAxisA=+Y  FollAlignAxisB=+Y  BaseAlignAxisB=+Z  RotationSequenceAxes=FollowerAxes  RotationSequence=XYX  RotationSequenceAngles=[0 0 0]  RotationSequenceAnglesUnits=deg  RotationMatrix=[1 0 0; 0 1 0; 0 0 1]
  DP Frame : PMIOPort  Side=Left
  MP Frame : PMIOPort  Port=2  Side=Left
  PP Frame : PMIOPort  Port=3  Side=Left
  CM AdAb : PMIOPort  Port=4  Side=Left
  connections:
  DIP Joint Shaft/RConn1 -- Distal Phalanx/LConn1 -- Revolute Joint1/RConn1
  Rigid Transform/LConn1 -- Middle Phalanx/LConn1
  Revolute Joint1/LConn1 -- Rigid Transform/RConn1
  DP Frame/RConn1 -- Distal Phalanx/RConn1
  MP Frame/RConn1 -- Middle Phalanx/RConn1
  PP Frame/RConn1 -- Proximal Phalanx/RConn1
  PIP Joint Shaft/RConn1 -- Middle Phalanx/LConn2 -- Revolute Joint/RConn1
  Rigid Transform1/LConn1 -- Proximal Phalanx/LConn1
  Revolute Joint/LConn1 -- Rigid Transform1/RConn1
  CM AdAb/RConn1 -- Proximal Phalanx/LConn2
